simulink model "q_cube"  (Simulink 7.8)
settings: Solver=FixedStepDiscrete  StartTime=0.0  StopTime=inf  FixedStep=0.002  MaxStep=10  RelTol=1e-3  AbsTol=1e-3
undefined symbols (not defined in the file): A11, A12, A21, A22, B1, B2, DiscIntNeverNeededParam, HIL, K, K_AMP, K_ENC, K_GYRO, L, qc_get_step_size, THETA_MAX, VMAX_AMP
libraries: quarc_library x6, simulink x2, simulink_extras x1
CloseFcn:
  | _discrete
settings Model: Creator=drmadill  LastModifiedBy=UCH  SimulationMode=external  ExtModeTrigDuration=50000  BufferReuse=off
settings SolverCC: PositivePriorityOrder=on
settings DataIOCC: LimitDataPoints=off  SaveOutput=off  SaveTime=off  SignalLoggingName=sigsOut
settings OptimizationCC: BooleanDataType=off  InlineInvariantSignals=on  OptimizeBlockIOStorage=off  BufferReuse=off  ExpressionFolding=off  LocalBlockOutputs=off  InitFltsAndDblsToZero=on
settings DebuggingCC: SaveWithParameterizedLinksMsg=none  SignalResolutionControl=TryResolveAllWithWarning  SolverPrmCheckMsg=none  MultiTaskDSMMsg=warning  MultiTaskCondExecSysMsg=none  FcnCallInpInsideContextMsg=Use local settings  StrictBusMsg=None
settings RTWCC: SystemTargetFile=quarc_win64.tlc  TemplateMakefile=quarc_default_tmf  Description=QUARC Win64 Target  ProcessScript=quarc_win64_make_rtw_hook
settings STFCustomTargetCC: TargetPreCompLibLocation=C:\PROGRA~3\QUARC\lib\2011b\win64\release  SystemTargetFile=quarc_win64.tlc
settings GRTTargetCC: TargetPreCompLibLocation=C:\PROGRA~3\QUARC\lib\2011b\win64\release  ParMdlRefBuildCompliant=off  CompOptLevelCompliant=off  ConcurrentExecutionCompliant=off  MatFileLogging=off  ExtMode=on  ExtModeMexFile=quarc_comm

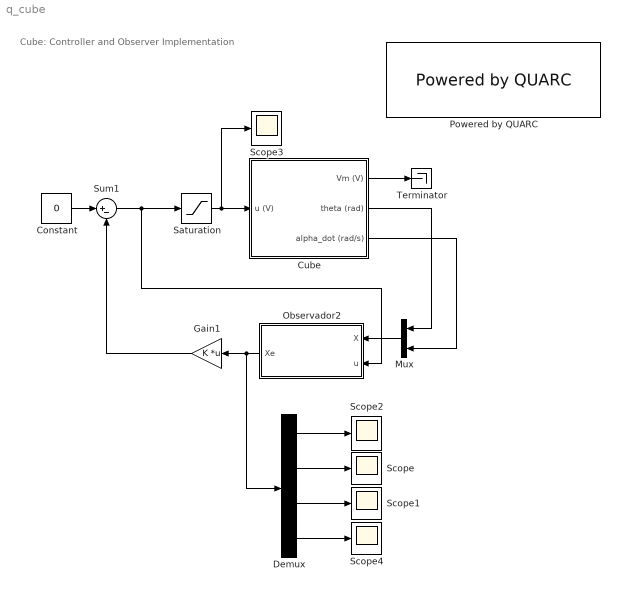
== system q_cube ==
  note: Cube: Controller and Observer Implementation
  Constant : Constant  Value=0
  Cube : Subsystem
  Demux : Demux
  Gain1 : Gain  Gain=K  Multiplication=Matrix(K*u)
  Mux : Mux  Inputs=2
  Observador2 : Subsystem
  Powered by QUARC : quarc_library/Logos/Powered by QUARC
  Saturation : Saturate  UpperLimit=0.2  LowerLimit=-0.2
  Scope{,1..4} (5 alike) : Scope
      Scope settings: YMin=-0.00625  YMax=-0.00375  SaveName=theta
      Scope1 settings: YMin=-0.025  YMax=0.0175  SaveName=alpha_dot
      Scope2 settings: YMin=-1.2e+307  YMax=4e+306  SaveName=alpha
      Scope3 settings: YMin=-4973506511820882200000000000000000000000000000000000000000000000000000000000000000000000000000.00000  YMax=1962907007491516200000000000000000000000000000000000000000000000000000000000000000000000000000.00000  SaveName=estados_lineal_discreto  DataFormat=Array
      Scope4 settings: YMin=-0.02  YMax=0.0175  SaveName=theta_dot
  Sum1 : Sum  Inputs=|+-
  Terminator : Terminator
  wires:
  Cube/2(theta (rad)) -> Mux/1
  Cube/3(alpha_dot (rad/s)) -> Mux/2
  Cube/1(Vm (V)) -> Terminator/1
  Constant/1 -> Sum1/1
  Sum1/1 -> Observador2/2(u), Saturation/1
  Mux/1 -> Observador2/1(X)
  Observador2/1(Xe) -> Gain1/1, Demux/1
  Gain1/1 -> Sum1/2
  Demux/3 -> Scope1/1
  Demux/2 -> Scope/1
  Demux/4 -> Scope4/1
  Demux/1 -> Scope2/1
  Saturation/1 -> Cube/1(u (V)), Scope3/1

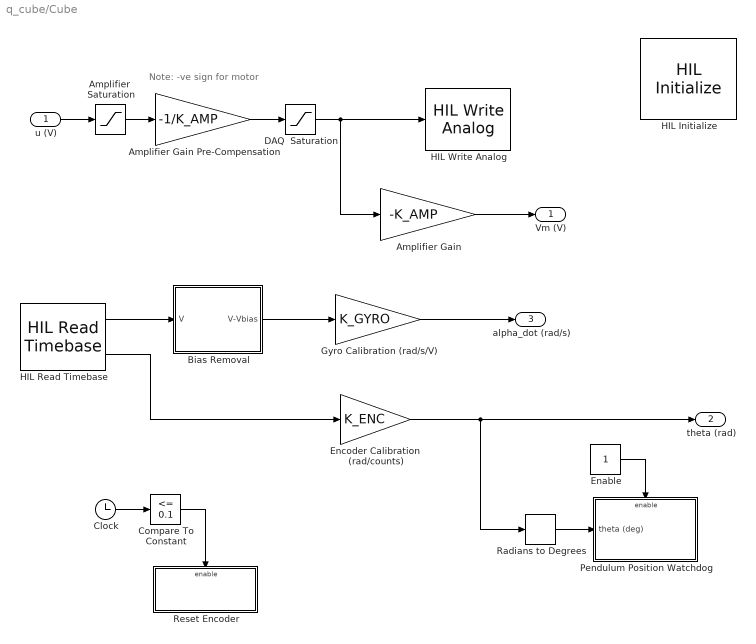
== system q_cube/Cube ==
  note: Note: -ve sign for motor
  u (V) : Inport
  Amplifier  Saturation : Saturate  UpperLimit=VMAX_AMP  LowerLimit=-VMAX_AMP
  Amplifier Gain : Gain  Gain=-K_AMP  SaturateOnIntegerOverflow=on  OutDataTypeStr=Inherit: Same as input  ParamDataTypeStr=Inherit: Same as input
  Amplifier Gain Pre-Compensation : Gain  Gain=-1/K_AMP  SaturateOnIntegerOverflow=on  OutDataTypeStr=Inherit: Same as input  ParamDataTypeStr=Inherit: Same as input
  Bias Removal : Subsystem  TreatAsAtomicUnit=on
  Clock : Clock
  Compare To Constant : simulink/Logic and Bit Operations/Compare To Constant  relop=<=  const=0.1  OutDataTypeStr=uint8  ZeroCross=off
  DAQ  Saturation : Saturate  UpperLimit=10  LowerLimit=-10
  Enable : Constant
  Encoder Calibration  (rad/counts) : Gain  Gain=K_ENC
  Gyro Calibration (rad/s/V) : Gain  Gain=K_GYRO  SaturateOnIntegerOverflow=on  OutDataTypeStr=Inherit: Same as input  ParamDataTypeStr=Inherit: Same as input
  HIL Initialize : quarc_library/Data Acquisition/Generic/Configuration/HIL Initialize  object_name=HIL-1  board_type=qpid  board_number=0  board_options=enc0_dir=0;enc0_filter=1;enc0_a=1;enc0_b=1;enc0_z=0;enc0_reload=0;enc1_dir=0;enc1_filter=1;enc1_a=1;enc1_b=1;enc1_z=0;enc1_reload=0;enc2_dir=0;enc2_filter=1;enc2_a=1;enc2_b=1;enc2_z=0;enc2_reload=0;enc3_dir=0;enc3_filter=1;enc3_a=1;enc3_b=1;enc3_z=0;enc3_reload=0;enc4_dir=0;enc4_filter=1;enc4_a=1;enc4_b=1;enc4_z=0;enc4_reload=0;enc5_dir=0;enc5_filter=1;enc5_a=1;enc5_b=1;enc5_z=0;enc5_reload=0;enc6_dir=0;enc6_filter=1;enc6_a=1;enc6_b=1;enc6_z=0;enc6_reload=0;enc7_dir=0;enc7_filter=1;enc7_a=1;enc7_b=1;enc7_z=0;enc7_reload=0;ext_int_polarity=0;fuse_polarity=0;convert_polarity=0;watchdog_polarity=0;ext_int_watchdog=0;fuse_watchdog=0;trig1_watchdog=0;watchdog_to_trig1=0;watchdog_to_trig2=0;counter_to_trig0=0;trigger_adcs=0;latch_on_adc=0;pwm_immediate=0  exclusive=off  active=on  hardware_clocks=[0:16]  clock_modes=[]  initial_clock_frequencies=[]  set_clock_params_at_start=off  set_clock_params_at_switch_in=off  set_clock_frequencies_at_start=off  set_clock_frequencies_at_switch_in=off  analog_input_channels=[0:7]  analog_input_maximums=10  analog_input_minimums=-10  set_analog_input_params_at_start=off  set_analog_input_params_at_switch_in=off  analog_output_channels=[0:7]  analog_output_maximums=10  analog_output_minimums=-10  initial_analog_outputs=[0]  final_analog_outputs=[0]  watchdog_analog_outputs=0  set_analog_output_params_at_start=off  set_analog_output_params_at_switch_in=off  set_analog_outputs_at_start=on  set_analog_outputs_at_switch_in=off  set_analog_outputs_at_terminate=on  set_analog_outputs_at_switch_out=off  set_analog_outputs_on_watchdog=off  digital_input_channels=[]  digital_output_channels=[]  digital_output_configuration=[]  initial_digital_outputs=[1]  final_digital_outputs=[1]  watchdog_digital_outputs=[2]  set_digital_output_params_at_start=off  set_digital_output_params_at_switch_in=off  set_digital_outputs_at_start=on  set_digital_outputs_at_switch_in=off  set_digital_outputs_at_terminate=on  set_digital_outputs_at_switch_out=off  set_digital_outputs_on_watchdog=off  encoder_channels=[0:7]  quadrature=[4]  encoder_filter_frequency=40e6/1  initial_encoder_counts=[0]  set_encoder_params_at_start=on  set_encoder_params_at_switch_in=off  set_encoder_counts_at_start=on  set_encoder_counts_at_switch_in=off  pwm_channels=[0:7]  pwm_modes=0  pwm_frequency=40e6/4096  pwm_configuration=[0]  pwm_alignment=[0]  pwm_polarity=[1]  pwm_leading_deadband=[0]  pwm_trailing_deadband=[0]  initial_pwm_outputs=[0]  final_pwm_outputs=[0]  watchdog_pwm_outputs=[0]  set_pwm_params_at_start=on  set_pwm_params_at_switch_in=off  set_pwm_outputs_at_start=on  set_pwm_outputs_at_switch_in=off  set_pwm_outputs_at_terminate=on  set_pwm_outputs_at_switch_out=off  set_pwm_outputs_on_watchdog=off  other_output_channels=[]  initial_other_outputs=[]  final_other_outputs=[]  watchdog_other_outputs=[]  set_other_outputs_at_start=off  set_other_outputs_at_switch_in=off  set_other_outputs_at_terminate=off  set_other_outputs_at_switch_out=off  set_other_outputs_on_watchdog=off
  HIL Read Timebase : quarc_library/Data Acquisition/Generic/Timebases/HIL Read Timebase  object_name=HIL-1  clock=0  analog_channels=1  encoder_channels=[0]  digital_channels=[]  other_channels=[]  samples_in_buffer=max(ceil(1/qc_get_step_size), 1)  active=on  vector_output=off  data_type_mode=Inherit via back propagation  encoder_data_type=double  digital_data_type=boolean
  HIL Write Analog : quarc_library/Data Acquisition/Generic/Immediate I//O/HIL Write Analog  object_name=HIL-1  channels=0  sample_time=-1  active=off  vector_input=off
  Pendulum Position Watchdog : Subsystem  TreatAsAtomicUnit=on
  Radians to Degrees : simulink_extras/Transformations/Radians to Degrees
  Reset Encoder : Subsystem  TreatAsAtomicUnit=on
  Vm (V) : Outport
  theta (rad) : Outport  Port=2
  alpha_dot (rad/s) : Outport  Port=3
  wires:
  Amplifier Gain Pre-Compensation/1 -> DAQ  Saturation/1
  Encoder Calibration  (rad/counts)/1 -> theta (rad)/1, Radians to Degrees/1
  Amplifier  Saturation/1 -> Amplifier Gain Pre-Compensation/1
  u (V)/1 -> Amplifier  Saturation/1
  HIL Read Timebase/2 -> Encoder Calibration  (rad/counts)/1
  Radians to Degrees/1 -> Pendulum Position Watchdog/1(theta (deg))
  Enable/1 -> Pendulum Position Watchdog/Enable
  Amplifier Gain/1 -> Vm (V)/1
  DAQ  Saturation/1 -> Amplifier Gain/1, HIL Write Analog/1
  HIL Read Timebase/1 -> Bias Removal/1(V)
  Bias Removal/1(V-Vbias) -> Gyro Calibration (rad/s/V)/1
  Clock/1 -> Compare To Constant/1
  Compare To Constant/1 -> Reset Encoder/Enable
  Gyro Calibration (rad/s/V)/1 -> alpha_dot (rad/s)/1

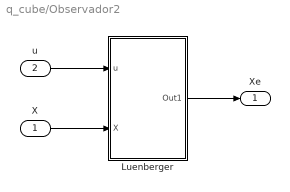
== system q_cube/Observador2 ==
  X : Inport
  u : Inport  Port=2
  Luenberger : Subsystem
  Xe : Outport
  wires:
  X/1 -> Luenberger/2(X)
  u/1 -> Luenberger/1(u)
  Luenberger/1(Out1) -> Xe/1

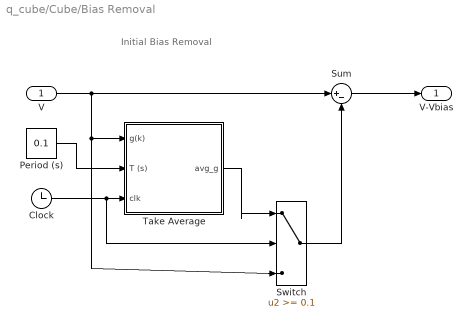
== system q_cube/Cube/Bias Removal ==
  note: Initial Bias Removal
  V : Inport
  Clock : Clock
  Period (s) : Constant  Value=0.1
  Sum : Sum  Inputs=|+-  SaturateOnIntegerOverflow=on  InputSameDT=on  OutDataTypeStr=Inherit: Same as first input
  Switch : Switch  Threshold=0.1
  Take Average : Subsystem
  V-Vbias : Outport
  wires:
  V/1 -> Sum/1, Take Average/1(g(k)), Switch/3
  Sum/1 -> V-Vbias/1
  Take Average/1(avg_g) -> Switch/1
  Switch/1 -> Sum/2
  Period (s)/1 -> Take Average/2(T (s))
  Clock/1 -> Take Average/3(clk), Switch/2

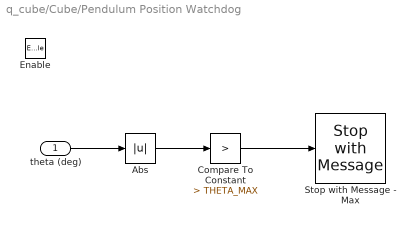
== system q_cube/Cube/Pendulum Position Watchdog ==
  theta (deg) : Inport
  Enable : EnablePort
  Abs : Abs
  Compare To Constant : simulink/Logic and Bit Operations/Compare To Constant  relop=>  const=THETA_MAX  OutDataTypeStr=uint8  ZeroCross=off
  Stop with Message - Max : quarc_library/Sinks/Error Handling/Stop with Message  message_type=Fixed error message  message_icon=Error  message=Pendulum reached maximum limit.
  wires:
  theta (deg)/1 -> Abs/1
  Abs/1 -> Compare To Constant/1
  Compare To Constant/1 -> Stop with Message - Max/1

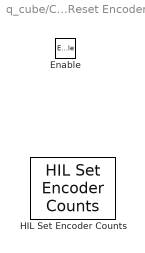
== system q_cube/Cube/Reset Encoder ==
  Enable : EnablePort
  HIL Set Encoder Counts : quarc_library/Data Acquisition/Generic/Configuration/HIL Set Encoder Counts  object_name=HIL-1  channels=0  source=internal  counts=0  sample_time=qc_get_step_size  active=on  vector_input=off
      settings: AttributesFormatString=(%<object_name>)

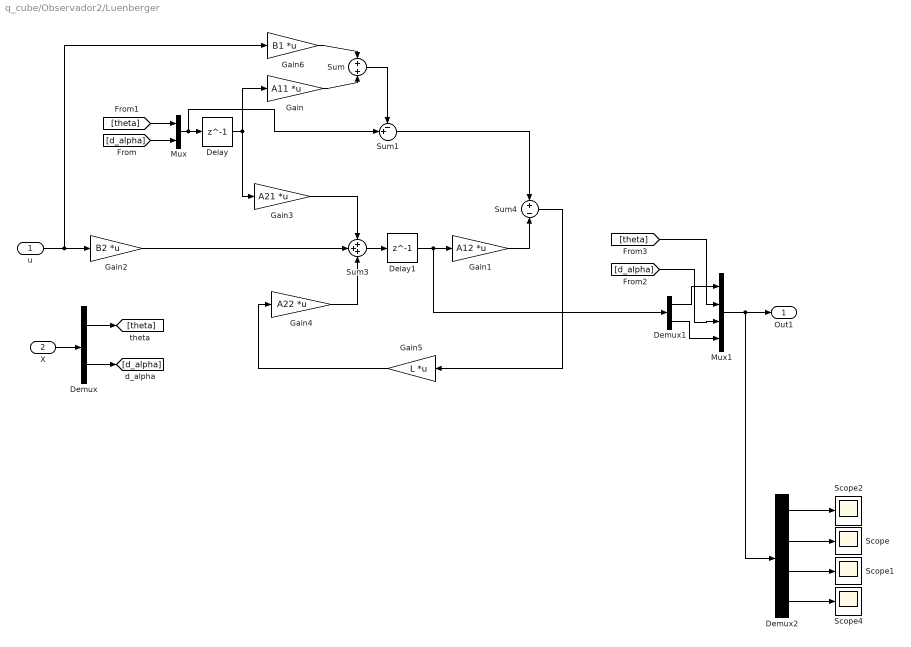
== system q_cube/Observador2/Luenberger ==
  u : Inport
  X : Inport  Port=2
  Delay : Delay  DelayLength=1
  Delay1 : Delay  DelayLength=1
  Demux : Demux  Outputs=2
  Demux1 : Demux  Outputs=2
  Demux2 : Demux
  Gain : Gain  Gain=A11  Multiplication=Matrix(K*u)
  Gain1 : Gain  Gain=A12  Multiplication=Matrix(K*u)
  Gain2 : Gain  Gain=B2  Multiplication=Matrix(K*u)
  Gain3 : Gain  Gain=A21  Multiplication=Matrix(K*u)
  Gain4 : Gain  Gain=A22  Multiplication=Matrix(K*u)
  Gain5 : Gain  Gain=L  Multiplication=Matrix(K*u)
  Gain6 : Gain  Gain=B1  Multiplication=Matrix(K*u)
  Mux : Mux  Inputs=2
  Mux1 : Mux
  Scope{,1..2,4} (4 alike) : Scope
      Scope settings: YMin=-0.00076699  YMax=-0.00076699  SaveName=theta1
      Scope1 settings: YMin=-0.02  YMax=0.0175  SaveName=alpha_dot1
      Scope2 settings: YMin=-1.2e+307  YMax=4e+306  SaveName=alpha1
      Scope4 settings: YMin=-0.02  YMax=0.0175  SaveName=theta_dot1
  Sum : Sum  Inputs=+|+
  Sum1 : Sum  Inputs=-+|
  Sum3 : Sum  Inputs=+++
  Sum4 : Sum  Inputs=+|-
  Out1 : Outport
  wires:
  Gain6/1 -> Sum/1
  Gain/1 -> Sum/2
  Sum4/1 -> Gain5/1
  u/1 -> Gain6/1, Gain2/1
  Gain2/1 -> Sum3/2
  Sum3/1 -> Delay1/1
  Mux1/1 -> Out1/1, Demux2/1
  Sum/1 -> Sum1/1
  X/1 -> Demux/1
  Gain3/1 -> Sum3/1
  Demux/2 -> [d_alpha]
  Demux/1 -> [theta]
  [d_alpha] -> Mux/2
  [theta] -> Mux/1
  Gain1/1 -> Sum4/2
  Sum1/1 -> Sum4/1
  Delay1/1 -> Gain1/1, Demux1/1
  Mux/1 -> Sum1/2, Delay/1
  Delay/1 -> Gain3/1, Gain/1
  Gain4/1 -> Sum3/3
  Demux1/1 -> Mux1/1
  [d_alpha] -> Mux1/3
  Demux1/2 -> Mux1/4
  [theta] -> Mux1/2
  Gain5/1 -> Gain4/1
  Demux2/3 -> Scope1/1
  Demux2/2 -> Scope/1
  Demux2/4 -> Scope4/1
  Demux2/1 -> Scope2/1

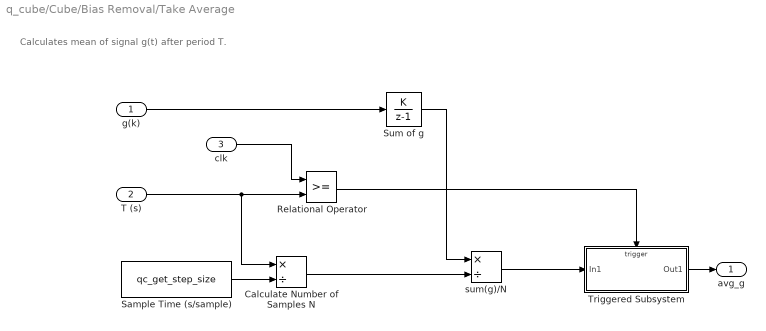
== system q_cube/Cube/Bias Removal/Take Average ==
  note: Calculates mean of signal g(t) after period T.
  g(k) : Inport
  T (s) : Inport  Port=2
  clk : Inport  Port=3
  Calculate Number of Samples N : Product  Inputs=*/
  Relational Operator : RelationalOperator  OutDataTypeStr=boolean
  Sample Time (s/sample) : Constant  Value=qc_get_step_size
  Sum of g : DiscreteIntegrator  IntegratorMethod=Accumulation: Forward Euler  SampleTime=qc_get_step_size  ICPrevOutput=DiscIntNeverNeededParam  ICPrevScaledInput=DiscIntNeverNeededParam
  Triggered Subsystem : Subsystem  TreatAsAtomicUnit=on
  sum(g)/N : Product  Inputs=*/
  avg_g : Outport
  wires:
  Triggered Subsystem/1(Out1) -> avg_g/1
  Sum of g/1 -> sum(g)/N/1
  sum(g)/N/1 -> Triggered Subsystem/1(In1)
  g(k)/1 -> Sum of g/1
  T (s)/1 -> Calculate Number of Samples N/1, Relational Operator/2
  Calculate Number of Samples N/1 -> sum(g)/N/2
  Sample Time (s/sample)/1 -> Calculate Number of Samples N/2
  Relational Operator/1 -> Triggered Subsystem/Trigger
  clk/1 -> Relational Operator/1

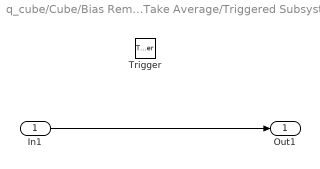
== system q_cube/Cube/Bias Removal/Take Average/Triggered Subsystem ==
  In1 : Inport
  Trigger : TriggerPort
  Out1 : Outport
  wires:
  In1/1 -> Out1/1
